simulink model "Model_05_Dynamic_RRF_PMSM_Model_and_FOC"  (R2020a)
settings: Solver=ode4  StartTime=0.0  StopTime=2  FixedStep=1e-4  RelTol=1e-3
InitFcn:
  | parameters_pmsm_ss
values from neighbouring files (symbols this model uses):
  Ki = BW*rs    (= 12.5663706144)    [parameters_pmsm_ss.m]
  Kp = BW*Lq    (= 0.0188495559215)    [parameters_pmsm_ss.m]
settings Model: Creator=samee  LastModifiedBy=DEVIKAT
settings DebuggingCC: UnconnectedInputMsg=none  UnconnectedOutputMsg=none  UnconnectedLineMsg=none

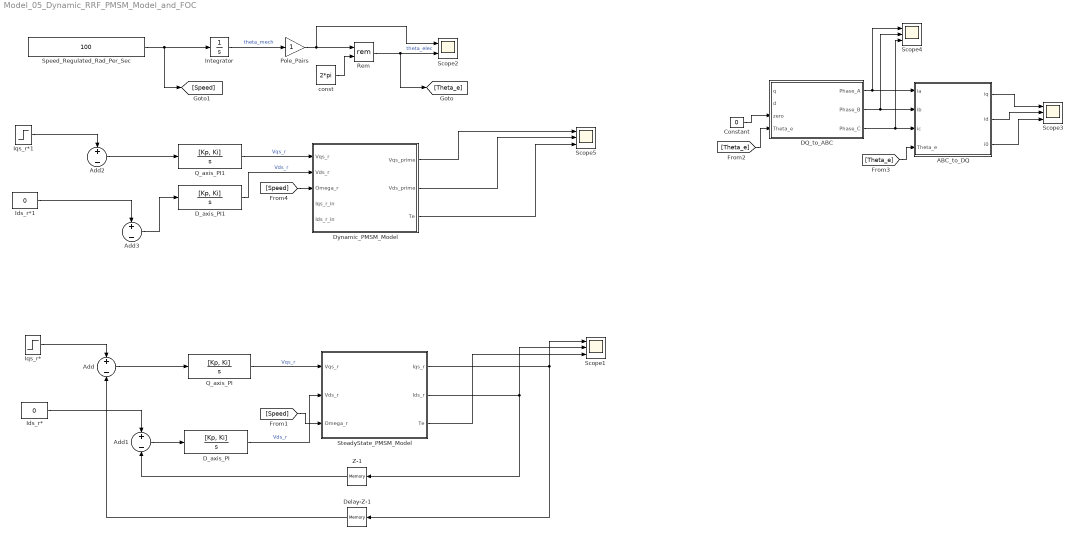
== system Model_05_Dynamic_RRF_PMSM_Model_and_FOC ==
  ABC_to_DQ : MATLAB Function  TreatAsAtomicUnit=on
  Add{,1..3} (4 alike) : Sum  Inputs=+-
  Constant : Constant  Value=0
  DQ_to_ABC : MATLAB Function  TreatAsAtomicUnit=on
  D_axis_PI : TransferFcn  Numerator=[Kp, Ki]  Denominator=[1 0]
  D_axis_PI1 : TransferFcn  Numerator=[Kp, Ki]  Denominator=[1 0]
  Delay-Z-1 : Memory
  Dynamic_PMSM_Model : MATLAB Function  TreatAsAtomicUnit=on
  Ids_r* : Constant  Value=0
  Ids_r*1 : Constant  Value=0
  Integrator : Integrator
  Iqs_r* : Step  After=2  SampleTime=0
  Iqs_r*1 : Step  After=2  SampleTime=0
  Pole_Pairs : Gain
  Q_axis_PI : TransferFcn  Numerator=[Kp, Ki]  Denominator=[1 0]
  Q_axis_PI1 : TransferFcn  Numerator=[Kp, Ki]  Denominator=[1 0]
  Rem : Math  Operator=rem  SaturateOnIntegerOverflow=on
  Scope{1,3..5} (4 alike) : Scope  NumInputPorts=3
  Scope2 : Scope  NumInputPorts=2
  Speed_Regulated_Rad_Per_Sec : Constant  Value=100
  SteadyState_PMSM_Model : MATLAB Function  TreatAsAtomicUnit=on
  Z-1 : Memory
  const : Constant  Value=2*pi
  wires:
  Integrator/1 -> Pole_Pairs/1  "theta_mech"
  const/1 -> Rem/2
  Pole_Pairs/1 -> Scope2/1, Rem/1
  Rem/1 -> Scope2/2, [Theta_e]  "theta_elec"
  Q_axis_PI/1 -> SteadyState_PMSM_Model/1(Vqs_r)  "Vqs_r"
  D_axis_PI/1 -> SteadyState_PMSM_Model/2(Vds_r)  "Vds_r"
  Speed_Regulated_Rad_Per_Sec/1 -> [Speed], Integrator/1
  [Speed] -> SteadyState_PMSM_Model/3(Omega_r)
  DQ_to_ABC/1(Phase_A) -> Scope4/1, ABC_to_DQ/1(ia)
  DQ_to_ABC/2(Phase_B) -> Scope4/2, ABC_to_DQ/2(ib)
  DQ_to_ABC/3(Phase_C) -> Scope4/3, ABC_to_DQ/3(ic)
  [Theta_e] -> DQ_to_ABC/4(Theta_e)
  Constant/1 -> DQ_to_ABC/3(zero)
  SteadyState_PMSM_Model/1(Iqs_r) -> Scope1/1, Delay-Z-1/1
  SteadyState_PMSM_Model/2(Ids_r) -> Scope1/2, Z-1/1
  SteadyState_PMSM_Model/3(Te) -> Scope1/3
  ABC_to_DQ/1(iq) -> Scope3/1
  ABC_to_DQ/2(id) -> Scope3/2
  ABC_to_DQ/3(i0) -> Scope3/3
  [Theta_e] -> ABC_to_DQ/4(Theta_e)
  Iqs_r*/1 -> Add/1
  Ids_r*/1 -> Add1/1
  Add/1 -> Q_axis_PI/1
  Add1/1 -> D_axis_PI/1
  Z-1/1 -> Add1/2
  Delay-Z-1/1 -> Add/2
  Add3/1 -> D_axis_PI1/1
  Add2/1 -> Q_axis_PI1/1
  Dynamic_PMSM_Model/3(Te) -> Scope5/3
  Dynamic_PMSM_Model/1(Vqs_prime) -> Scope5/1
  Ids_r*1/1 -> Add3/1
  D_axis_PI1/1 -> Dynamic_PMSM_Model/2(Vds_r)  "Vds_r"
  Dynamic_PMSM_Model/2(Vds_prime) -> Scope5/2
  [Speed] -> Dynamic_PMSM_Model/3(Omega_r)
  Iqs_r*1/1 -> Add2/1
  Q_axis_PI1/1 -> Dynamic_PMSM_Model/1(Vqs_r)  "Vqs_r"

== matlab function Model_05_Dynamic_RRF_PMSM_Model_and_FOC/DQ_to_ABC ==
  data: q input; d input; Phase_A output; zero input; Theta_e input; Phase_B output; Phase_C output
function [Phase_A, Phase_B, Phase_C] = fcn(q, d, zero, Theta_e)

Phase_A = cos(Theta_e)*q + sin(Theta_e)*d + zero*1;
Phase_B = cos(Theta_e-(2*pi/3))*q + sin(Theta_e-(2*pi/3))*d + zero*1;
Phase_C = cos(Theta_e+(2*pi/3))*q + sin(Theta_e+(2*pi/3))*d + zero*1;

== matlab function Model_05_Dynamic_RRF_PMSM_Model_and_FOC/SteadyState_PMSM_Model ==
  data: Vqs_r input; Vds_r input; Omega_r input; Iqs_r output; Ids_r output; Te output
function [Iqs_r, Ids_r, Te] = SS_PMSM_Model(Vqs_r, Vds_r, Omega_r)
%#codegen

rs = 0.2;               %Stator resistance
Lq = 300e-6;            %d and q axis inductances
Ld = 300e-6;
Lambda_m_r = 0.01;      %rotor flux linkages (back-emf constant)
P=2;                    % numer of poles   


K1 = ((rs^2) + (Omega_r^2)*Ld*Lq);

% Motor currents in rotor reference frame
Iqs_r = (rs/K1) * (Vqs_r - Omega_r*Lambda_m_r - (Omega_r*Ld/rs)*Vds_r);
Ids_r = (1/K1) * (rs*Vds_r + Omega_r*Lq*Vqs_r - (Omega_r^2)*Lq*Lambda_m_r);

% Electromagnetic torque generated
Te = (3/2)*(P/2)*((Lambda_m_r*Iqs_r) + ((Ld - Lq)*Iqs_r*Ids_r));

== matlab function Model_05_Dynamic_RRF_PMSM_Model_and_FOC/ABC_to_DQ ==
  data: ia input; ib input; iq output; ic input; Theta_e input; id output; i0 output
function [iq, id, i0] = fcn(ia, ib, ic, Theta_e)
%#codegen
% Ks    =   (2/3)*[ cos(Theta_e)        cos(Theta_e-(2*pi/3))           cos(Theta_e+(2*pi/3));
%                   sin (Theta_e)       sin (Theta_e-(2*pi/3))          sin(Theta_e+(2*pi/3));
%                   0.5                 0.5                             0.5 ];
% 
% iqd0  =   Ks*[ia;ib;ic];
% 
% iq    =   iqd0(1);
% id    =   iqd0(2);
% 10    =   iqd0(3);

iq = (2/3)*(cos(Theta_e)*ia + cos(Theta_e-(2*pi/3))*ib + cos(Theta_e+(2*pi/3))*ic); 
id = (2/3)*(sin(Theta_e)*ia + sin(Theta_e-(2*pi/3))*ib + sin(Theta_e+(2*pi/3))*ic); 
i0 = (2/3)*(0.5*ia + 0.5*ib + 0.5*ic);

== matlab function Model_05_Dynamic_RRF_PMSM_Model_and_FOC/Dynamic_PMSM_Model ==
  data: Vqs_r input; Vds_r input; Omega_r input; Iqs_r_in input; Ids_r_in input; Vqs_prime output; Vds_prime output; Te output
function [Vqs_prime, Vds_prime, Te] = fcn(Vqs_r, Vds_r, Omega_r, Iqs_r_in, Ids_r_in)

rs          = 0.2;      %Stator resistance
Lq          = 300e-6;   %d and q axis inductances
Ld          = 300e-6;
Lambda_m_r  = 0.01;     %rotor flux linkages (back-emf constant)
P           = 2;        %poles


Vqs_prime   = (Vqs_r - Omega_r*Lambda_m_r - Omega_r*Ld*Ids_r_in);
Vds_prime   = (Vds_r + Omega_r*Lq*Iqs_r_in);


Te = (3/2)*(P/2)*(Lambda_m_r*Iqs_r_in +(Ld-Lq)*Iqs_r_in*Ids_r_in);
